simulink model "ExampleModel"  (R2024b)
settings: Solver=VariableStepAuto  StartTime=0.0  StopTime=10.0  RelTol=1e-3
libraries: simulink x3
settings Model: Creator=nikola  LastModifiedBy=nikola

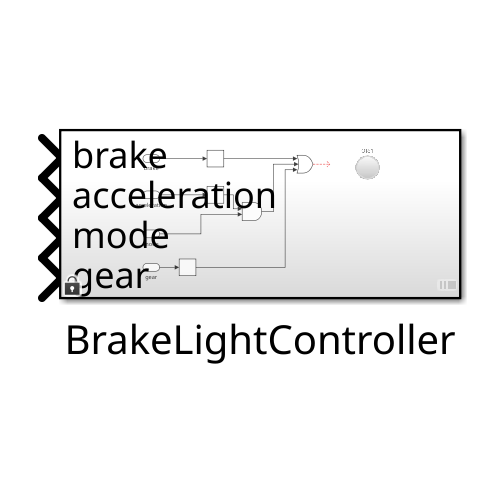
[thumbnail: Simulink's stored preview of the top-level diagram]
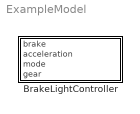
== system ExampleModel ==
  BrakeLightController : Subsystem

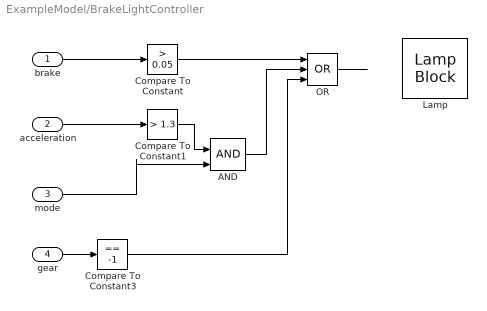
== system ExampleModel/BrakeLightController ==
  brake : Inport
  acceleration : Inport  Port=2
  mode : Inport  Port=3
  gear : Inport  Port=4
  AND : Logic  IconShape=distinctive  AllPortsSameDT=off  OutDataTypeStr=boolean
  Compare To Constant : simulink/Logic and Bit Operations/Compare To Constant  relop=>  const=0.05  OutDataTypeStr=boolean
  Compare To Constant1 : simulink/Logic and Bit Operations/Compare To Constant  relop=>  const=1.3  OutDataTypeStr=boolean
  Compare To Constant3 : simulink/Logic and Bit Operations/Compare To Constant  relop===  const=-1  OutDataTypeStr=boolean
  Lamp : LampBlock
  OR : Logic  Operator=OR  Inputs=3  IconShape=distinctive  AllPortsSameDT=off  OutDataTypeStr=boolean
  wires:
  brake/1 -> Compare To Constant/1
  acceleration/1 -> Compare To Constant1/1
  mode/1 -> AND/2
  Compare To Constant1/1 -> AND/1
  AND/1 -> OR/2
  OR/1 -> ?
  Compare To Constant/1 -> OR/1
  gear/1 -> Compare To Constant3/1
  Compare To Constant3/1 -> OR/3
